simulink model "sine_wave_iir_12bit"  (Simulink 6.6)
settings: Solver=VariableStepDiscrete  SolverMode=SingleTasking  StartTime=0.0  StopTime=16384/100e6  RelTol=1e-3
StopFcn:
  | doFFTPlot(100e6,[IIRDiscr,IIRD2FT(:,1:16385)'],['IIRDiscr';'IIRD2FT '],1,1,'hann')
undefined symbols (not defined in the file): dfilt
libraries: xbsIndex_r4 x9, dsparch4 x1, dspsrcs4 x1
settings Model: Creator=lcrockett  LastModifiedBy=lcrockett
settings DataIOCC: SignalLoggingName=sigsOut
settings OptimizationCC: InlineParams=on  InlineInvariantSignals=on
settings DebuggingCC: SignalResolutionControl=TryResolveAllWithWarning  SolverPrmCheckMsg=none  MultiTaskDSMMsg=warning  MultiTaskCondExecSysMsg=none  StrictBusMsg=None
settings HardwareCC: TargetUnknown=on
settings RTWCC: IncludeERTFirstTime=on
settings GRTTargetCC: ModelReferenceCompliant=off  MatFileLogging=off

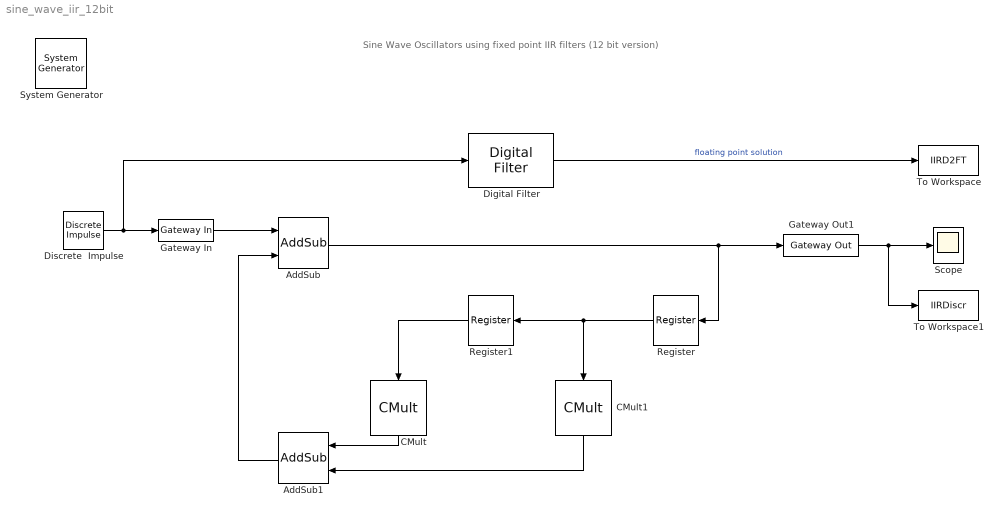
== system sine_wave_iir_12bit ==
  note: Sine Wave Oscillators using fixed point IIR filters (12 bit version)
  " System Generator" : xbsIndex_r4/ System Generator  Tag=genX  SystemSampleTime=-1  xilinxfamily=virtex2p  part=xc2vp30  speed=-7  package=ff896  synthesis_tool=XST  clock_wrapper=Clock Enables  directory=./netlist  testbench=off  simulink_period=1/100e6  sysclk_period=50  dcm_input_clock_period=100  incr_netlist=off  trim_vbits=Everywhere in SubSystem  dbl_ovrd=According to Block Masks  core_generation=According to Block Masks  run_coregen=off  deprecated_control=off  eval_field=0  block_type=sysgen
      settings: block_version=9.2.01
  AddSub : xbsIndex_r4/AddSub  mode=Addition  use_carryin=off  use_carryout=off  en=off  latency=0  precision=User Defined  arith_type="Signed  (2's comp)"  n_bits=12  bin_pt=9  quantization="Round  (unbiased: +/- Inf)"  overflow=Wrap  dbl_ovrd=off  use_behavioral_HDL=on  pipelined=off  use_rpm=on  block_type=addsub
      settings: xl_area=[0, 0, 0, 0, 0, 0, 0]  block_version=VER_STRING_GOES_HERE
  AddSub1 : xbsIndex_r4/AddSub  Orientation=left  mode=Addition  use_carryin=off  use_carryout=off  en=off  latency=0  precision=User Defined  arith_type="Signed  (2's comp)"  n_bits=12  bin_pt=9  quantization=Truncate  overflow=Wrap  dbl_ovrd=off  use_behavioral_HDL=on  pipelined=off  use_rpm=on  block_type=addsub
      settings: xl_area=[0, 0, 0, 0, 0, 0, 0]  block_version=VER_STRING_GOES_HERE
  CMult : xbsIndex_r4/CMult  Orientation=down  const=-1  const_n_bits=2  const_bin_pt=0  en=off  latency=0  precision=User Defined  arith_type="Signed  (2's comp)"  n_bits=12  bin_pt=9  quantization="Round  (unbiased: +/- Inf)"  overflow=Wrap  dbl_ovrd=off  use_behavioral_HDL=off  mem_type=Distributed RAM  placement_style=Rectangular Shape  pipeline=off  use_rpm=on  block_type=cmult
      settings: xl_area=[0, 0, 0, 0, 0, 0, 0]  block_version=VER_STRING_GOES_HERE
  CMult1 : xbsIndex_r4/CMult  Orientation=down  const=1.75  const_n_bits=4  const_bin_pt=2  en=off  latency=0  precision=User Defined  arith_type="Signed  (2's comp)"  n_bits=12  bin_pt=9  quantization="Round  (unbiased: +/- Inf)"  overflow=Flag as error  dbl_ovrd=off  use_behavioral_HDL=off  mem_type=Distributed RAM  placement_style=Rectangular Shape  pipeline=off  use_rpm=on  block_type=cmult
      settings: xl_area=[0, 0, 0, 0, 0, 0, 0]  block_version=VER_STRING_GOES_HERE
  Digital Filter : dsparch4/Digital Filter  DialogController=dspdialog.DigitalFilter  DialogControllerArgs=DataTag1  TypePopup=IIR (poles & zeros)  IIRFiltStruct=Direct form II transposed  AllPoleFiltStruct=Direct form  FIRFiltStruct=Direct form  CoeffSource=Specify via dialog  NumCoeffs=[1]  DenCoeffs=[1 -1.75 1]  BiQuadCoeffs=[1 0.3 0.4 1 0.1 0.2]  LatticeCoeffs=[0.2 0.4]  denIgnore=on  FiltPerSampPopup=One filter per frame  IC=0  ICnum=0  ICden=0  roundingMode=Floor  overflowMode=off  ScaleValues=1  scaleValueFracLength=14  stageInFracLength=15  stageOutFracLength=15  FilterSource=Specify via dialog  dfiltObjectName=dfilt.dffir([1 2 1])
  Discrete  Impulse : dspsrcs4/Discrete  Impulse  Delay=0  SampleTime=1/100e6  FrameSample=1  dataType=double  isSigned=on  wordLen=16  udDataType=sfix(16)  fracBitsMode=Best precision  numFracBits=14
  Gateway In : xbsIndex_r4/Gateway In  arith_type="Signed  (2's comp)"  n_bits=12  bin_pt=10  quantization=Truncate  overflow=Wrap  period=1/100e6  dbl_ovrd=off  timing_constraint=None  locs_specified=off  LOCs={}  block_type=gatewayin
      settings: infoedit="Gateway in block.  Converts inputs of type Simulink integer, double and fixed point to  Xilinx fixed point type.<P><P>Hardware notes:  In hardware these blocks become top level input ports."  xl_area=[0, 0, 0, 0, 0, 0, 0]  block_version=VER_STRING_GOES_HERE
  Gateway Out1 : xbsIndex_r4/Gateway Out  hdl_port=on  timing_constraint=None  locs_specified=off  LOCs={}  block_type=gatewayout
      settings: infoedit="Gateway out block.  Converts Xilinx fixed point inputs into ouputs of type Simulink integer, double, or fixed point.<P><P>Hardware notes:  In hardware these blocks become top level output ports or are discarded, depending on how they are configured."  xl_area=[0, 0, 0, 0, 0, 0, 0]  block_version=VER_STRING_GOES_HERE
  Register : xbsIndex_r4/Register  Orientation=left  init=0  rst=off  en=off  dbl_ovrd=off  block_type=register
      settings: xl_area=[0, 0, 0, 0, 0, 0, 0]  block_version=VER_STRING_GOES_HERE
  Register1 : xbsIndex_r4/Register  Orientation=left  init=0  rst=off  en=off  dbl_ovrd=off  block_type=register
      settings: xl_area=[0, 0, 0, 0, 0, 0, 0]  block_version=VER_STRING_GOES_HERE
  Scope : Scope
      settings: TimeRange=9.836065573770391e-007  YMin=-2.5  YMax=2.5
  To Workspace : ToWorkspace  VariableName=IIRD2FT  SampleTime=-1  SaveFormat=Array
  To Workspace1 : ToWorkspace  VariableName=IIRDiscr  SampleTime=-1  SaveFormat=Array
  wires:
  Gateway In/1 -> AddSub/1
  AddSub/1 -> Register/1, Gateway Out1/1
  Register/1 -> Register1/1, CMult1/1
  CMult/1 -> AddSub1/1
  Gateway Out1/1 -> Scope/1, To Workspace1/1
  CMult1/1 -> AddSub1/2
  AddSub1/1 -> AddSub/2
  Register1/1 -> CMult/1
  Discrete  Impulse/1 -> Gateway In/1, Digital Filter/1
  Digital Filter/1 -> To Workspace/1  "floating point solution"
